simulink model "Skematik_Pagi_R2024b0x2Daziz"  (R2024b)
settings: Solver=ode23tb  StartTime=0.0  StopTime=2  RelTol=1e-3
undefined symbols (not defined in the file): D1, Delta
libraries: spsThreePhaseBreakerLib x87, spsThreePhaseParallelRLCLoadLib x19, spsThreePhaseTransformerTwoWindingsLib x18, spsThreePhasePISectionLineLib x18, spsExcitationSystemLib x4, spsSynchronousMachinepuStandardLib x4, spsThreePhaseVIMeasurementLib x4, spsMultimeterLib x1, spspowerguiLib x1
settings Model: Creator=Rafi Ananta Alden  LastModifiedBy=Ahmad Aziz

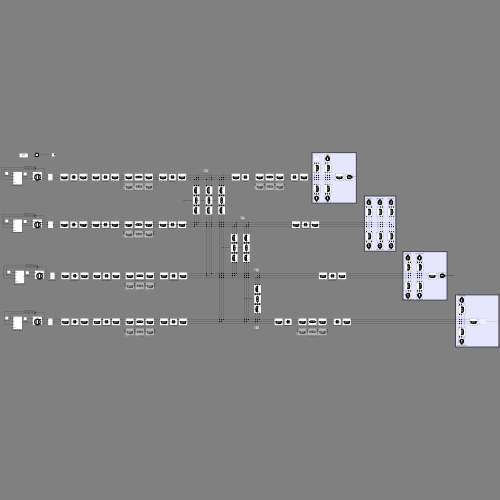
[thumbnail: Simulink's stored preview of the top-level diagram]
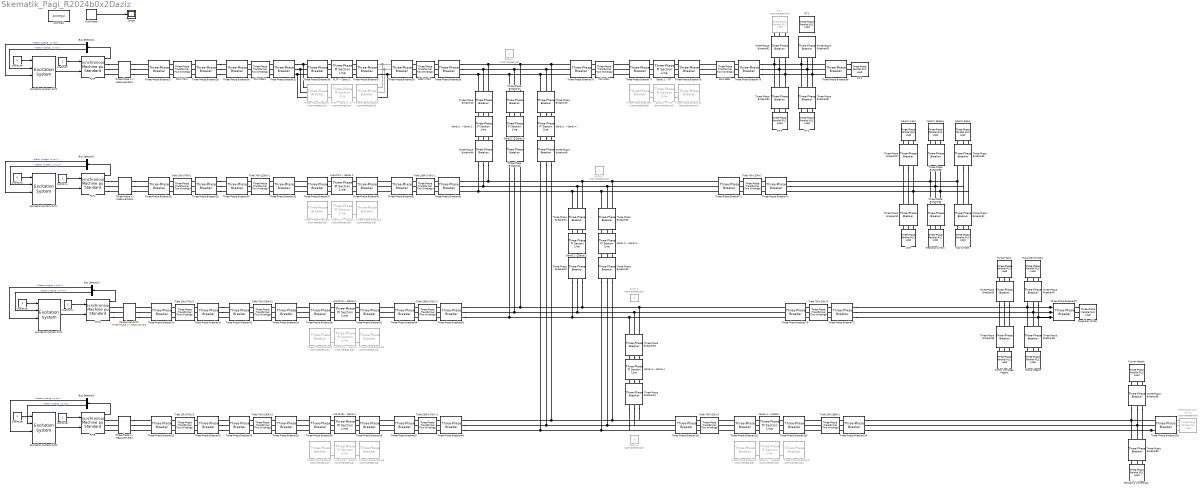
== system Skematik_Pagi_R2024b0x2Daziz ==
  20kV/380V : spsThreePhaseTransformerTwoWindingsLib/Three-Phase Transformer (Two Windings)  Winding1Connection=Yg  Winding2Connection=Delta (D1)  CoreType=Three single-phase transformers  SetSaturation=off  Hysteresis=off  DataFile='hysteresis'  SetInitialFlux=off  Measurements=None  UNITS=pu  NominalPower=[ 1000e6 , 50 ]  Winding1=[ 20e3 , 5e-3 , 0.1/(100*pi) ]  Winding2=[ 380 , 5e-3 , 0 ]  Rm=500  Lm=500  L0=0.5  Saturation=[ 0,0 ; 0.0024,1.2 ; 1.0,1.52 ]  InitialFluxes=[ 0.8 , -0.8 , 0.7 ]  BreakLoop=off  DiscreteSolver=Trapezoidal iterative  DataType=off  TransfoNumber=1
  20kV/70kV : spsThreePhaseTransformerTwoWindingsLib/Three-Phase Transformer (Two Windings)  Winding1Connection=Yg  Winding2Connection=Delta (D1)  CoreType=Three single-phase transformers  SetSaturation=off  Hysteresis=off  DataFile='hysteresis'  SetInitialFlux=off  Measurements=None  UNITS=pu  NominalPower=[ 250e6 , 50 ]  Winding1=[ 20e3 , 0.005 , 0 ]  Winding2=[ 70e3 , 0.005 , 0.1/314 ]  Rm=500  Lm=500  L0=0.5  Saturation=[ 0,0 ; 0.0024,1.2 ; 1.0,1.52 ]  InitialFluxes=[ 0.8 , -0.8 , 0.7 ]  BreakLoop=off  DiscreteSolver=Trapezoidal iterative  DataType=off  TransfoNumber=1
  "230kV/70kV " : spsThreePhaseTransformerTwoWindingsLib/Three-Phase Transformer (Two Windings)  Winding1Connection=Yg  Winding2Connection=Delta (D1)  CoreType=Three single-phase transformers  SetSaturation=off  Hysteresis=off  DataFile='hysteresis'  SetInitialFlux=off  Measurements=None  UNITS=pu  NominalPower=[ 250e6 , 50 ]  Winding1=[ 230e3 , 5e-3 , 0.1/(100*pi) ]  Winding2=[ 70e3 , 5e-3 , 0 ]  Rm=500  Lm=500  L0=0.5  Saturation=[ 0,0 ; 0.0024,1.2 ; 1.0,1.52 ]  InitialFluxes=[ 0.8 , -0.8 , 0.7 ]  BreakLoop=off  DiscreteSolver=Trapezoidal iterative  DataType=off  TransfoNumber=1
  70kV/20kV : spsThreePhaseTransformerTwoWindingsLib/Three-Phase Transformer (Two Windings)  Winding1Connection=Delta (D1)  Winding2Connection=Yg  CoreType=Three single-phase transformers  SetSaturation=off  Hysteresis=off  DataFile='hysteresis'  SetInitialFlux=off  Measurements=None  UNITS=pu  NominalPower=[ 250e6 , 50 ]  Winding1=[70e3 , 0.005 , 0.1/314 ]  Winding2=[ 20e3 , 0.005 , 0 ]  Rm=500  Lm=500  L0=0.5  Saturation=[ 0,0 ; 0.0024,1.2 ; 1.0,1.52 ]  InitialFluxes=[ 0.8 , -0.8 , 0.7 ]  BreakLoop=off  DiscreteSolver=Trapezoidal iterative  DataType=off  TransfoNumber=1
  70kV/230kV : spsThreePhaseTransformerTwoWindingsLib/Three-Phase Transformer (Two Windings)  Winding1Connection=Delta (D1)  Winding2Connection=Yg  CoreType=Three single-phase transformers  SetSaturation=off  Hysteresis=off  DataFile='hysteresis'  SetInitialFlux=off  Measurements=None  UNITS=pu  NominalPower=[ 250e6 , 50 ]  Winding1=[ 70e3 , 5e-3 , 0.1/(100*pi) ]  Winding2=[ 230e3 , 5e-3 , 0 ]  Rm=500  Lm=500  L0=0.5  Saturation=[ 0,0 ; 0.0024,1.2 ; 1.0,1.52 ]  InitialFluxes=[ 0.8 , -0.8 , 0.7 ]  BreakLoop=off  DiscreteSolver=Trapezoidal iterative  DataType=off  TransfoNumber=1
  Bus Selector{1..4} (4 alike) : BusSelector  OutputSignals="dq0 components.Stator voltage  vq (pu),dq0 components.Stator voltage  vd (pu)"
  Excitation System PLTA : spsExcitationSystemLib/Excitation System  tr=20e-3  reg=[ 300, 0.001 ]  exc=[ 1, 0 ]  tgr=[ 0, 0 ]  damp=[ 0.001, 0.1 ]  sat=[ 0, 0 ]  lim=[ -11.5, 11.5, 0 ]  v0="[1.0  1.28]"
      settings: LibrarySourceBlock=sps_lib/Electrical Machines/Synchronous Machine Control/Excitation System
  Excitation System PLTB : spsExcitationSystemLib/Excitation System  tr=20e-3  reg=[ 300, 0.001 ]  exc=[ 1, 0 ]  tgr=[ 0, 0 ]  damp=[ 0.001, 0.1 ]  sat=[ 0, 0 ]  lim=[ -11.5, 11.5, 0 ]  v0="[1.0  1.28]"
      settings: LibrarySourceBlock=sps_lib/Electrical Machines/Synchronous Machine Control/Excitation System
  Excitation System PLTP : spsExcitationSystemLib/Excitation System  tr=20e-3  reg=[ 300, 0.001 ]  exc=[ 1, 0 ]  tgr=[ 0, 0 ]  damp=[ 0.001, 0.1 ]  sat=[ 0, 0 ]  lim=[ -11.5, 11.5, 0 ]  v0="[1.0  1.28]"
      settings: LibrarySourceBlock=sps_lib/Electrical Machines/Synchronous Machine Control/Excitation System
  Excitation System PLTU : spsExcitationSystemLib/Excitation System  tr=20e-3  reg=[ 300, 0.001 ]  exc=[ 1, 0 ]  tgr=[ 0, 0 ]  damp=[ 0.001, 0.1 ]  sat=[ 0, 0 ]  lim=[ -11.5, 11.5, 0 ]  v0="[1.0  1.28]"
      settings: LibrarySourceBlock=sps_lib/Electrical Machines/Synchronous Machine Control/Excitation System
  Gardu 1 : Constant  Commented=on
  "Gardu 1 -- Gardu 2" : spsThreePhasePISectionLineLib/Three-Phase PI Section Line  LConnTagsString=a|b|c  RConnTagsString=A|B|C  Length=20  Frequency=50  Resistances=[ 0.2 0.2]  Inductances="[ 0.00637  0.00637]"  Capacitances=[12.74e-9 7.751e-9]
  "Gardu 1 -- Gardu 3" : spsThreePhasePISectionLineLib/Three-Phase PI Section Line  LConnTagsString=a|b|c  RConnTagsString=A|B|C  Length=5  Frequency=50  Resistances=[ 0.2 0.2]  Inductances="[ 0.00637  0.00637]"  Capacitances=[12.74e-9 7.751e-9]
  "Gardu 1 -- Gardu 4" : spsThreePhasePISectionLineLib/Three-Phase PI Section Line  LConnTagsString=a|b|c  RConnTagsString=A|B|C  Length=20  Frequency=50  Resistances=[ 0.2 0.2]  Inductances="[ 0.00637  0.00637]"  Capacitances=[12.74e-9 7.751e-9]
  "Gardu 1 -- RT" : spsThreePhasePISectionLineLib/Three-Phase PI Section Line  LConnTagsString=a|b|c  RConnTagsString=A|B|C  Length=3  Frequency=50  Resistances=[ 0.2 0.2]  Inductances="[ 0.00637  0.00637]"  Capacitances=[12.74e-9 7.751e-9]
  "Gardu 1 -- RT1" : spsThreePhasePISectionLineLib/Three-Phase PI Section Line  Commented=on  LConnTagsString=a|b|c  RConnTagsString=A|B|C  Length=3  Frequency=50  Resistances=[0.05 0.25]  Inductances=[0.001 0.003]  Capacitances=[10e-9 7e-9]
  Gardu 2 : Constant  Commented=on  Value=2
  "Gardu 2 -- Gardu 3" : spsThreePhasePISectionLineLib/Three-Phase PI Section Line  LConnTagsString=a|b|c  RConnTagsString=A|B|C  Length=5  Frequency=50  Resistances=[ 0.2 0.2]  Inductances="[ 0.00637  0.00637]"  Capacitances=[12.74e-9 7.751e-9]
  "Gardu 2 -- Gardu 4" : spsThreePhasePISectionLineLib/Three-Phase PI Section Line  LConnTagsString=a|b|c  RConnTagsString=A|B|C  Length=20  Frequency=50  Resistances=[ 0.2 0.2]  Inductances="[ 0.00637  0.00637]"  Capacitances=[12.74e-9 7.751e-9]
  Gardu 3 : Constant  Commented=on  Value=3
  "Gardu 3 -- Gardu 4" : spsThreePhasePISectionLineLib/Three-Phase PI Section Line  LConnTagsString=a|b|c  RConnTagsString=A|B|C  Length=5  Frequency=50  Resistances=[ 0.2 0.2]  Inductances="[ 0.00637  0.00637]"  Capacitances=[12.74e-9 7.751e-9]
  Gardu 4 : Constant  Commented=on  Value=4
  "Gardu 4 -- PubSos" : spsThreePhasePISectionLineLib/Three-Phase PI Section Line  LConnTagsString=a|b|c  RConnTagsString=A|B|C  Length=3  Frequency=50  Resistances=[ 0.1 0.1]  Inductances="[ 0.00637  0.00637]"  Capacitances=[12.74e-9 7.751e-9]
  "Gardu 4 -- PubSos1" : spsThreePhasePISectionLineLib/Three-Phase PI Section Line  Commented=on  LConnTagsString=a|b|c  RConnTagsString=A|B|C  Length=3  Frequency=50  Resistances=[0.05 0.25]  Inductances=[0.001 0.003]  Capacitances=[10e-9 7e-9]
  Industri Besar : spsThreePhaseParallelRLCLoadLib/Three-Phase Parallel RLC Load  LConnTagsString=A|B|C  Configuration=Y (grounded)  NominalVoltage=20e3  Vabc=[1e3 1e3 1e3]  Vabcp=[1e3 1e3 1e3]  NominalFrequency=50  UnbalancedPower=off  ActivePower=9.00e6  InductivePower=4.36e6  CapacitivePower=0  Pabc=[10e3 9e3 11e3]  QLabc=[100 90 110]  QCabc=[100 90 110]  Pabcp=[10e3 9e3 11e3]  QLabcp=[100 90 110]  QCabcp=[100 90 110]  Measurements=Branch voltages and currents  LoadType=constant Z
  Industri Kecil : spsThreePhaseParallelRLCLoadLib/Three-Phase Parallel RLC Load  LConnTagsString=A|B|C  Configuration=Y (grounded)  NominalVoltage=20e3  Vabc=[1e3 1e3 1e3]  Vabcp=[1e3 1e3 1e3]  NominalFrequency=50  UnbalancedPower=off  ActivePower=5.94e9  InductivePower=2.88e9  CapacitivePower=0  Pabc=[10e3 9e3 11e3]  QLabc=[100 90 110]  QCabc=[100 90 110]  Pabcp=[10e3 9e3 11e3]  QLabcp=[100 90 110]  QCabcp=[100 90 110]  Measurements=Branch voltages and currents  LoadType=constant Z
  Industri Sedang : spsThreePhaseParallelRLCLoadLib/Three-Phase Parallel RLC Load  LConnTagsString=A|B|C  Configuration=Y (grounded)  NominalVoltage=20e3  Vabc=[1e3 1e3 1e3]  Vabcp=[1e3 1e3 1e3]  NominalFrequency=50  UnbalancedPower=off  ActivePower=4.50e7  InductivePower=2.18e7  CapacitivePower=0  Pabc=[10e3 9e3 11e3]  QLabc=[100 90 110]  QCabc=[100 90 110]  Pabcp=[10e3 9e3 11e3]  QLabcp=[100 90 110]  QCabcp=[100 90 110]  Measurements=Branch voltages and currents  LoadType=constant Z
  Istana Negara : spsThreePhaseParallelRLCLoadLib/Three-Phase Parallel RLC Load  LConnTagsString=A|B|C  Configuration=Y (grounded)  NominalVoltage=20e3  Vabc=[1e3 1e3 1e3]  Vabcp=[1e3 1e3 1e3]  NominalFrequency=50  UnbalancedPower=off  ActivePower=1.17e6  InductivePower=5.67e5  CapacitivePower=0  Pabc=[10e3 9e3 11e3]  QLabc=[100 90 110]  QCabc=[100 90 110]  Pabcp=[10e3 9e3 11e3]  QLabcp=[100 90 110]  QCabcp=[100 90 110]  Measurements=Branch voltages and currents  LoadType=constant Z
  Kantor Lembaga Negara : spsThreePhaseParallelRLCLoadLib/Three-Phase Parallel RLC Load  LConnTagsString=A|B|C  Configuration=Y (grounded)  NominalVoltage=20e3  Vabc=[1e3 1e3 1e3]  Vabcp=[1e3 1e3 1e3]  NominalFrequency=50  UnbalancedPower=off  ActivePower=1.80e6  InductivePower=8.72e5  CapacitivePower=0  Pabc=[10e3 9e3 11e3]  QLabc=[100 90 110]  QCabc=[100 90 110]  Pabcp=[10e3 9e3 11e3]  QLabcp=[100 90 110]  QCabcp=[100 90 110]  Measurements=Branch voltages and currents  LoadType=constant Z
  "Line PLTA -- Gardu 1" : spsThreePhasePISectionLineLib/Three-Phase PI Section Line  Commented=on  LConnTagsString=a|b|c  RConnTagsString=A|B|C  Length=50  Frequency=50  Resistances=[ 0.2 0.3864]  Inductances="[ 2/(100*pi)  4.1264e-3]"  Capacitances=[12.74e-9 7.751e-9]
  "Line PLTA -- Gardu 3" : spsThreePhasePISectionLineLib/Three-Phase PI Section Line  LConnTagsString=a|b|c  RConnTagsString=A|B|C  Length=50  Frequency=50  Resistances=[ 0.2 0.3864]  Inductances="[ 2/(100*pi)  4.1264e-3]"  Capacitances=[12.74e-9 7.751e-9]
  "Line PLTB -- Gardu 1" : spsThreePhasePISectionLineLib/Three-Phase PI Section Line  Commented=on  LConnTagsString=a|b|c  RConnTagsString=A|B|C  Length=20  Frequency=50  Resistances=[ 0.2 0.3864]  Inductances="[ 2/(100*pi)  4.1264e-3]"  Capacitances=[12.74e-9 7.751e-9]
  "Line PLTB -- Gardu 4" : spsThreePhasePISectionLineLib/Three-Phase PI Section Line  LConnTagsString=a|b|c  RConnTagsString=A|B|C  Length=20  Frequency=50  Resistances=[ 0.2 0.3864]  Inductances="[ 2/(100*pi)  4.1264e-3]"  Capacitances=[12.74e-9 7.751e-9]
  "Line PLTU -- Gardu 1" : spsThreePhasePISectionLineLib/Three-Phase PI Section Line  Commented=on  LConnTagsString=a|b|c  RConnTagsString=A|B|C  Length=100  Frequency=50  Resistances=[0.05 0.25]  Inductances=[0.001 0.003]  Capacitances=[10e-9 7e-9]
  "Line PLTU -- Gardu 2" : spsThreePhasePISectionLineLib/Three-Phase PI Section Line  LConnTagsString=a|b|c  RConnTagsString=A|B|C  Length=100  Frequency=50  Resistances=[ 0.2 0.2]  Inductances="[ 0.00637  0.00637]"  Capacitances=[12.74e-9 7.751e-9]
  Mall & Hotel : spsThreePhaseParallelRLCLoadLib/Three-Phase Parallel RLC Load  LConnTagsString=A|B|C  Configuration=Y (grounded)  NominalVoltage=20e3  Vabc=[1e3 1e3 1e3]  Vabcp=[1e3 1e3 1e3]  NominalFrequency=50  UnbalancedPower=off  ActivePower=9.00e5  InductivePower=4.36e5  CapacitivePower=0  Pabc=[10e3 9e3 11e3]  QLabc=[100 90 110]  QCabc=[100 90 110]  Pabcp=[10e3 9e3 11e3]  QLabcp=[100 90 110]  QCabcp=[100 90 110]  Measurements=Branch voltages and currents  LoadType=constant Z
  Multimeter : spsMultimeterLib/Multimeter  L=108  sel=1  yselected={}  Gain=0  OutputType=Magnitude  PlotAtSimulationStop=off  PhasorSimulation=on
  PLTA : spsSynchronousMachinepuStandardLib/Synchronous Machine pu Standard  PresetModel=No  MechanicalLoad=Mechanical power Pm  ShowDetailedParameters=on  RotorType=Salient-pole  Units=per unit standard parameters  MeasurementBus=off  NominalParameters="[34e6  20e3   50]"  Reactances1=[ 1.81, 0.3, 0.23, 1.76, 0.65, 0.25, 0.15 ]  Reactances2="[1.305, 0.296, 0.252, 0.474,  0.243,  0.1]"  dAxisTimeConstants=Open-circuit  qAxisTimeConstants=Short-circuit  TimeConstants1="[ 4.4849  0.0681  0.1  ]"  TimeConstants2=[ 8.0, 0.03, 1.0, 0.07 ]  TimeConstants3="[  4.49  0.0681  0.0513  ]"  TimeConstants4=[ 8.0, 0.03, 0.3371, 0.0295 ]  TimeConstants5=[ 1.01, 0.053, 0.1 ]  TimeConstants6=[ 1.3201, 0.023, 1.0, 0.07 ]  TimeConstants7=[0.012 0.003 0.003]  TimeConstants8=[ 1.3201, 0.0231, 0.3371, 0.0295 ]  StatorResistance=0.003  Mechanical=[3.7 0 20]  PolePairs=20  InitialConditions=[0 -84.041 0.282629 0.282629 0.282629 44.9561 -75.0439 164.956 0.763822]  SetSaturation=off  Saturation=[0.6404,0.7127,0.8441,0.9214,0.9956,1.082,1.19,1.316,1.457;0.7,0.7698,0.8872,0.9466,0.9969,1.046,1.1,1.151,1.201]  LoadFlowParameters=[1,0,0,0,0]  TsPowergui=0  TsBlock=-1  IterativeModel=Trapezoidal non iterative  IterativeDiscreteModel=Trapezoidal non iterative  BusType=swing  Pref=100e6*1  Qref=0  Qmin=-100e6  Qmax=100e6  PLF=0  QLF=0
  PLTB : spsSynchronousMachinepuStandardLib/Synchronous Machine pu Standard  PresetModel=No  MechanicalLoad=Mechanical power Pm  ShowDetailedParameters=on  RotorType=Salient-pole  Units=per unit standard parameters  MeasurementBus=off  NominalParameters="[11e6  20e3   50]"  Reactances1=[ 1.81, 0.3, 0.23, 1.76, 0.65, 0.25, 0.15 ]  Reactances2="[1.305, 0.296, 0.252, 0.474,  0.243,  0.1]"  dAxisTimeConstants=Open-circuit  qAxisTimeConstants=Short-circuit  TimeConstants1="[ 4.4849  0.0681  0.1  ]"  TimeConstants2=[ 8.0, 0.03, 1.0, 0.07 ]  TimeConstants3="[  4.49  0.0681  0.0513  ]"  TimeConstants4=[ 8.0, 0.03, 0.3371, 0.0295 ]  TimeConstants5=[ 1.01, 0.053, 0.1 ]  TimeConstants6=[ 1.3201, 0.023, 1.0, 0.07 ]  TimeConstants7=[0.012 0.003 0.003]  TimeConstants8=[ 1.3201, 0.0231, 0.3371, 0.0295 ]  StatorResistance=0.003  Mechanical=[3.7 0 20]  PolePairs=20  InitialConditions=[0 -84.041 0.282629 0.282629 0.282629 44.9561 -75.0439 164.956 0.763822]  SetSaturation=off  Saturation=[0.6404,0.7127,0.8441,0.9214,0.9956,1.082,1.19,1.316,1.457;0.7,0.7698,0.8872,0.9466,0.9969,1.046,1.1,1.151,1.201]  LoadFlowParameters=[1,0,0,0,0]  TsPowergui=0  TsBlock=-1  IterativeModel=Trapezoidal non iterative  IterativeDiscreteModel=Trapezoidal non iterative  BusType=PV  Pref=100e6*1  Qref=0  Qmin=-100e6  Qmax=100e6  PLF=0  QLF=0
  "PLTP " : spsSynchronousMachinepuStandardLib/Synchronous Machine pu Standard  PresetModel=No  MechanicalLoad=Mechanical power Pm  ShowDetailedParameters=on  RotorType=Salient-pole  Units=per unit standard parameters  MeasurementBus=off  NominalParameters="[89e6  20e3   50]"  Reactances1=[ 1.81, 0.3, 0.23, 1.76, 0.65, 0.25, 0.15 ]  Reactances2="[1.305, 0.296, 0.252, 0.474,  0.243,  0.1]"  dAxisTimeConstants=Open-circuit  qAxisTimeConstants=Short-circuit  TimeConstants1="[ 4.4849  0.0681  0.1  ]"  TimeConstants2=[ 8.0, 0.03, 1.0, 0.07 ]  TimeConstants3="[  4.49  0.0681  0.0513  ]"  TimeConstants4=[ 8.0, 0.03, 0.3371, 0.0295 ]  TimeConstants5=[ 1.01, 0.053, 0.1 ]  TimeConstants6=[ 1.3201, 0.023, 1.0, 0.07 ]  TimeConstants7=[0.012 0.003 0.003]  TimeConstants8=[ 1.3201, 0.0231, 0.3371, 0.0295 ]  StatorResistance=0.003  Mechanical=[3.7 0 20]  PolePairs=20  InitialConditions=[0 -87.2037 0.333145 0.333145 0.333145 75.164 -44.836 195.164 0.584783]  SetSaturation=off  Saturation=[0.6404,0.7127,0.8441,0.9214,0.9956,1.082,1.19,1.316,1.457;0.7,0.7698,0.8872,0.9466,0.9969,1.046,1.1,1.151,1.201]  LoadFlowParameters=[1,0,0,0,0]  TsPowergui=0  TsBlock=-1  IterativeModel=Trapezoidal non iterative  IterativeDiscreteModel=Trapezoidal non iterative  BusType=swing  Pref=0  Qref=0  Qmin=-inf  Qmax=inf  PLF=0  QLF=0
  "PLTP -- Gardu 1" : spsThreePhasePISectionLineLib/Three-Phase PI Section Line  LConnTagsString=a|b|c  RConnTagsString=A|B|C  Length=100  Frequency=50  Resistances=[ 0.2 0.2]  Inductances="[ 0.00637  0.00637]"  Capacitances=[12.74e-9 7.751e-9]
  "PLTP -- Gardu 1 (1)" : spsThreePhasePISectionLineLib/Three-Phase PI Section Line  Commented=on  LConnTagsString=a|b|c  RConnTagsString=A|B|C  Length=100  Frequency=50  Resistances=[0.05 0.25]  Inductances=[0.001 0.003]  Capacitances=[10e-9 7e-9]
  PLTU : spsSynchronousMachinepuStandardLib/Synchronous Machine pu Standard  PresetModel=No  MechanicalLoad=Mechanical power Pm  ShowDetailedParameters=on  RotorType=Salient-pole  Units=per unit standard parameters  MeasurementBus=off  NominalParameters="[111e6  20e3   50]"  Reactances1=[ 1.81, 0.3, 0.23, 1.76, 0.65, 0.25, 0.15 ]  Reactances2="[1.305, 0.296, 0.252, 0.474,  0.243,  0.1]"  dAxisTimeConstants=Open-circuit  qAxisTimeConstants=Short-circuit  TimeConstants1="[ 4.4849  0.0681  0.1  ]"  TimeConstants2=[ 8.0, 0.03, 1.0, 0.07 ]  TimeConstants3="[  4.49  0.0681  0.0513  ]"  TimeConstants4=[ 8.0, 0.03, 0.3371, 0.0295 ]  TimeConstants5=[ 1.01, 0.053, 0.1 ]  TimeConstants6=[ 1.3201, 0.023, 1.0, 0.07 ]  TimeConstants7=[0.012 0.003 0.003]  TimeConstants8=[ 1.3201, 0.0231, 0.3371, 0.0295 ]  StatorResistance=0.003  Mechanical=[3.7 0 20]  PolePairs=20  InitialConditions=[0 -84.041 0.282629 0.282629 0.282629 44.9561 -75.0439 164.956 0.763822]  SetSaturation=off  Saturation=[0.6404,0.7127,0.8441,0.9214,0.9956,1.082,1.19,1.316,1.457;0.7,0.7698,0.8872,0.9466,0.9969,1.046,1.1,1.151,1.201]  LoadFlowParameters=[1,0,0,0,0]  TsPowergui=0  TsBlock=-1  IterativeModel=Trapezoidal non iterative  IterativeDiscreteModel=Trapezoidal non iterative  BusType=PV  Pref=82e6  Qref=0  Qmin=-100e6  Qmax=100e6  PLF=0  QLF=0
  Pangkalan Militer : spsThreePhaseParallelRLCLoadLib/Three-Phase Parallel RLC Load  LConnTagsString=A|B|C  Configuration=Y (grounded)  NominalVoltage=20e3  Vabc=[1e3 1e3 1e3]  Vabcp=[1e3 1e3 1e3]  NominalFrequency=50  UnbalancedPower=off  ActivePower=1.35e4  InductivePower=6.54e3  CapacitivePower=0  Pabc=[10e3 9e3 11e3]  QLabc=[100 90 110]  QCabc=[100 90 110]  Pabcp=[10e3 9e3 11e3]  QLabcp=[100 90 110]  QCabcp=[100 90 110]  Measurements=Branch voltages and currents  LoadType=constant Z
  Penerangan Jalan Umum : spsThreePhaseParallelRLCLoadLib/Three-Phase Parallel RLC Load  Commented=on  LConnTagsString=A|B|C  Configuration=Y (grounded)  NominalVoltage=20e3  Vabc=[1e3 1e3 1e3]  Vabcp=[1e3 1e3 1e3]  NominalFrequency=50  UnbalancedPower=off  ActivePower=0  InductivePower=0  CapacitivePower=0  Pabc=[10e3 9e3 11e3]  QLabc=[100 90 110]  QCabc=[100 90 110]  Pabcp=[10e3 9e3 11e3]  QLabcp=[100 90 110]  QCabcp=[100 90 110]  Measurements=Branch voltages and currents  LoadType=constant Z
  Pengukuran PLTA : spsThreePhaseVIMeasurementLib/Three-Phase V-I Measurement  VoltageMeasurement=phase-to-ground  SetLabelV=on  LabelV=V_PLTA  Vpu=off  VpuLL=off  CurrentMeasurement=yes  SetLabelI=on  LabelI=I_PLTA  Ipu=off  Pbase=100e6  Vbase=500e3  OutputType=Complex  PhasorSimulation=on  PSBequivalent=0
  Pref PLTA : Constant
  Pref PLTB : Constant
  Pref PLTP : Constant
  Pref PLTU : Constant
  Pusat Server Data : spsThreePhaseParallelRLCLoadLib/Three-Phase Parallel RLC Load  LConnTagsString=A|B|C  Configuration=Y (grounded)  NominalVoltage=20e3  Vabc=[1e3 1e3 1e3]  Vabcp=[1e3 1e3 1e3]  NominalFrequency=50  UnbalancedPower=off  ActivePower=2.25e5  InductivePower=1.09e5  CapacitivePower=0  Pabc=[10e3 9e3 11e3]  QLabc=[100 90 110]  QCabc=[100 90 110]  Pabcp=[10e3 9e3 11e3]  QLabcp=[100 90 110]  QCabcp=[100 90 110]  Measurements=Branch voltages and currents  LoadType=constant Z
  RT 1 : spsThreePhaseParallelRLCLoadLib/Three-Phase Parallel RLC Load  Commented=on  LConnTagsString=A|B|C  Configuration=Y (grounded)  NominalVoltage=20e3  Vabc=[1e3 1e3 1e3]  Vabcp=[1e3 1e3 1e3]  NominalFrequency=50  UnbalancedPower=off  ActivePower=0  InductivePower=0  CapacitivePower=0  Pabc=[10e3 9e3 11e3]  QLabc=[100 90 110]  QCabc=[100 90 110]  Pabcp=[10e3 9e3 11e3]  QLabcp=[100 90 110]  QCabcp=[100 90 110]  Measurements=Branch voltages and currents  LoadType=constant Z
  RT 2 : spsThreePhaseParallelRLCLoadLib/Three-Phase Parallel RLC Load  LConnTagsString=A|B|C  Configuration=Y (grounded)  NominalVoltage=20e3  Vabc=[1e3 1e3 1e3]  Vabcp=[1e3 1e3 1e3]  NominalFrequency=50  UnbalancedPower=off  ActivePower=8e6  InductivePower=3.87e6  CapacitivePower=0  Pabc=[10e3 9e3 11e3]  QLabc=[100 90 110]  QCabc=[100 90 110]  Pabcp=[10e3 9e3 11e3]  QLabcp=[100 90 110]  QCabcp=[100 90 110]  Measurements=Branch voltages and currents  LoadType=constant Z
  RT 3 : spsThreePhaseParallelRLCLoadLib/Three-Phase Parallel RLC Load  LConnTagsString=A|B|C  Configuration=Y (grounded)  NominalVoltage=20e3  Vabc=[1e3 1e3 1e3]  Vabcp=[1e3 1e3 1e3]  NominalFrequency=50  UnbalancedPower=off  ActivePower=5.10e6  InductivePower=2.47e6  CapacitivePower=0  Pabc=[10e3 9e3 11e3]  QLabc=[100 90 110]  QCabc=[100 90 110]  Pabcp=[10e3 9e3 11e3]  QLabcp=[100 90 110]  QCabcp=[100 90 110]  Measurements=Branch voltages and currents  LoadType=constant Z
  RT 4 : spsThreePhaseParallelRLCLoadLib/Three-Phase Parallel RLC Load  LConnTagsString=A|B|C  Configuration=Y (grounded)  NominalVoltage=20e3  Vabc=[1e3 1e3 1e3]  Vabcp=[1e3 1e3 1e3]  NominalFrequency=50  UnbalancedPower=off  ActivePower=2.10e6  InductivePower=1.02e6  CapacitivePower=0  Pabc=[10e3 9e3 11e3]  QLabc=[100 90 110]  QCabc=[100 90 110]  Pabcp=[10e3 9e3 11e3]  QLabcp=[100 90 110]  QCabcp=[100 90 110]  Measurements=Branch voltages and currents  LoadType=constant Z
  RT 5 : spsThreePhaseParallelRLCLoadLib/Three-Phase Parallel RLC Load  LConnTagsString=A|B|C  Configuration=Y (grounded)  NominalVoltage=20e3  Vabc=[1e3 1e3 1e3]  Vabcp=[1e3 1e3 1e3]  NominalFrequency=50  UnbalancedPower=off  ActivePower=3.60e6  InductivePower=1.74e6  CapacitivePower=0  Pabc=[10e3 9e3 11e3]  QLabc=[100 90 110]  QCabc=[100 90 110]  Pabcp=[10e3 9e3 11e3]  QLabcp=[100 90 110]  QCabcp=[100 90 110]  Measurements=Branch voltages and currents  LoadType=constant Z
  Restoran & Toko : spsThreePhaseParallelRLCLoadLib/Three-Phase Parallel RLC Load  LConnTagsString=A|B|C  Configuration=Y (grounded)  NominalVoltage=20e3  Vabc=[1e3 1e3 1e3]  Vabcp=[1e3 1e3 1e3]  NominalFrequency=50  UnbalancedPower=off  ActivePower=4.50e6  InductivePower=2.18e6  CapacitivePower=0  Pabc=[10e3 9e3 11e3]  QLabc=[100 90 110]  QCabc=[100 90 110]  Pabcp=[10e3 9e3 11e3]  QLabcp=[100 90 110]  QCabcp=[100 90 110]  Measurements=Branch voltages and currents  LoadType=constant Z
  Rumah Ibadah : spsThreePhaseParallelRLCLoadLib/Three-Phase Parallel RLC Load  LConnTagsString=A|B|C  Configuration=Y (grounded)  NominalVoltage=20e3  Vabc=[1e3 1e3 1e3]  Vabcp=[1e3 1e3 1e3]  NominalFrequency=50  UnbalancedPower=off  ActivePower=5.94e9  InductivePower=2.88e9  CapacitivePower=0  Pabc=[10e3 9e3 11e3]  QLabc=[100 90 110]  QCabc=[100 90 110]  Pabcp=[10e3 9e3 11e3]  QLabcp=[100 90 110]  QCabcp=[100 90 110]  Measurements=Branch voltages and currents  LoadType=constant Z
  Rumah Sakit : spsThreePhaseParallelRLCLoadLib/Three-Phase Parallel RLC Load  LConnTagsString=A|B|C  Configuration=Y (grounded)  NominalVoltage=20e3  Vabc=[1e3 1e3 1e3]  Vabcp=[1e3 1e3 1e3]  NominalFrequency=50  UnbalancedPower=off  ActivePower=3.96e7  InductivePower=1.92e7  CapacitivePower=0  Pabc=[10e3 9e3 11e3]  QLabc=[100 90 110]  QCabc=[100 90 110]  Pabcp=[10e3 9e3 11e3]  QLabcp=[100 90 110]  QCabcp=[100 90 110]  Measurements=Branch voltages and currents  LoadType=constant Z
  Scope : Scope
  Sekolah & Universitas : spsThreePhaseParallelRLCLoadLib/Three-Phase Parallel RLC Load  LConnTagsString=A|B|C  Configuration=Y (grounded)  NominalVoltage=20e3  Vabc=[1e3 1e3 1e3]  Vabcp=[1e3 1e3 1e3]  NominalFrequency=50  UnbalancedPower=off  ActivePower=4.50e7  InductivePower=2.18e7  CapacitivePower=0  Pabc=[10e3 9e3 11e3]  QLabc=[100 90 110]  QCabc=[100 90 110]  Pabcp=[10e3 9e3 11e3]  QLabcp=[100 90 110]  QCabcp=[100 90 110]  Measurements=Branch voltages and currents  LoadType=constant Z
  Three-Phase V-I Measurement1 : spsThreePhaseVIMeasurementLib/Three-Phase V-I Measurement  VoltageMeasurement=phase-to-ground  SetLabelV=on  LabelV=V_PLTU  Vpu=off  VpuLL=off  CurrentMeasurement=yes  SetLabelI=on  LabelI=I_PLTU  Ipu=off  Pbase=100e6  Vbase=500e3  OutputType=Magnitude  PhasorSimulation=on  PSBequivalent=0
  Three-Phase V-I Measurement2 : spsThreePhaseVIMeasurementLib/Three-Phase V-I Measurement  VoltageMeasurement=phase-to-ground  SetLabelV=on  LabelV=V_PLTB  Vpu=off  VpuLL=off  CurrentMeasurement=yes  SetLabelI=on  LabelI=I_PLTB  Ipu=off  Pbase=100e6  Vbase=500e3  OutputType=Complex  PhasorSimulation=on  PSBequivalent=0
  Three-Phase V-I Measurement4 : spsThreePhaseVIMeasurementLib/Three-Phase V-I Measurement  VoltageMeasurement=phase-to-ground  SetLabelV=on  LabelV=V_PLTP  Vpu=off  VpuLL=off  CurrentMeasurement=yes  SetLabelI=on  LabelI=I_PLTP  Ipu=off  Pbase=100e6  Vbase=500e3  OutputType=Complex  PhasorSimulation=on  PSBequivalent=0
  Three-Phase Breaker{1..12} (12 alike) : spsThreePhaseBreakerLib/Three-Phase Breaker  Commented=on  InitialState=closed  SwitchA=on  SwitchB=on  SwitchC=on  SwitchTimes="[0.4  1.3]"  External=off  BreakerResistance=0.01  SnubberResistance=1e6  SnubberCapacitance=inf  Measurements=None
  Three-Phase Breaker{24..67,70..73,76..79,82..104} (75 alike) : spsThreePhaseBreakerLib/Three-Phase Breaker  InitialState=closed  SwitchA=on  SwitchB=on  SwitchC=on  SwitchTimes="[0.4  1.3]"  External=off  BreakerResistance=0.01  SnubberResistance=1e6  SnubberCapacitance=inf  Measurements=None
  Trafo 20kV/380V1 : spsThreePhaseTransformerTwoWindingsLib/Three-Phase Transformer (Two Windings)  Winding1Connection=Yg  Winding2Connection=Delta (D1)  CoreType=Three single-phase transformers  SetSaturation=off  Hysteresis=off  DataFile='hysteresis'  SetInitialFlux=off  Measurements=None  UNITS=pu  NominalPower=[ 1000e6 , 50 ]  Winding1=[ 20e3 , 5e-3 , 0.1/(100*pi) ]  Winding2=[ 380 , 5e-3 , 0 ]  Rm=500  Lm=500  L0=0.5  Saturation=[ 0,0 ; 0.0024,1.2 ; 1.0,1.52 ]  InitialFluxes=[ 0.8 , -0.8 , 0.7 ]  BreakLoop=off  DiscreteSolver=Trapezoidal iterative  DataType=off  TransfoNumber=1
  Trafo 20kV/70kV1 : spsThreePhaseTransformerTwoWindingsLib/Three-Phase Transformer (Two Windings)  Winding1Connection=Yg  Winding2Connection=Delta (D1)  CoreType=Three single-phase transformers  SetSaturation=off  Hysteresis=off  DataFile='hysteresis'  SetInitialFlux=off  Measurements=None  UNITS=pu  NominalPower=[ 250e6 , 50 ]  Winding1=[ 20e3 , 0.005 , 0 ]  Winding2=[ 70e3 , 0.005 , 0.1/314 ]  Rm=500  Lm=500  L0=0.5  Saturation=[ 0,0 ; 0.0024,1.2 ; 1.0,1.52 ]  InitialFluxes=[ 0.8 , -0.8 , 0.7 ]  BreakLoop=off  DiscreteSolver=Trapezoidal iterative  DataType=off  TransfoNumber=1
  Trafo 20kV/70kV2 : spsThreePhaseTransformerTwoWindingsLib/Three-Phase Transformer (Two Windings)  Winding1Connection=Yg  Winding2Connection=Delta (D1)  CoreType=Three single-phase transformers  SetSaturation=off  Hysteresis=off  DataFile='hysteresis'  SetInitialFlux=off  Measurements=None  UNITS=pu  NominalPower=[ 250e6 , 50 ]  Winding1=[ 20e3 , 0.005 , 0 ]  Winding2=[ 70e3 , 0.005 , 0.1/314 ]  Rm=500  Lm=500  L0=0.5  Saturation=[ 0,0 ; 0.0024,1.2 ; 1.0,1.52 ]  InitialFluxes=[ 0.8 , -0.8 , 0.7 ]  BreakLoop=off  DiscreteSolver=Trapezoidal iterative  DataType=off  TransfoNumber=1
  Trafo 20kV/70kV3 : spsThreePhaseTransformerTwoWindingsLib/Three-Phase Transformer (Two Windings)  Winding1Connection=Yg  Winding2Connection=Delta (D1)  CoreType=Three single-phase transformers  SetSaturation=off  Hysteresis=off  DataFile='hysteresis'  SetInitialFlux=off  Measurements=None  UNITS=pu  NominalPower=[ 250e6 , 50 ]  Winding1=[ 20e3 , 0.005 , 0 ]  Winding2=[ 70e3 , 0.005 , 0.1/314 ]  Rm=500  Lm=500  L0=0.5  Saturation=[ 0,0 ; 0.0024,1.2 ; 1.0,1.52 ]  InitialFluxes=[ 0.8 , -0.8 , 0.7 ]  BreakLoop=off  DiscreteSolver=Trapezoidal iterative  DataType=off  TransfoNumber=1
  Trafo 230kV/70kV 1 : spsThreePhaseTransformerTwoWindingsLib/Three-Phase Transformer (Two Windings)  Winding1Connection=Yg  Winding2Connection=Delta (D1)  CoreType=Three single-phase transformers  SetSaturation=off  Hysteresis=off  DataFile='hysteresis'  SetInitialFlux=off  Measurements=None  UNITS=pu  NominalPower=[ 250e6 , 50 ]  Winding1=[ 20e3 , 5e-3 , 0.1/(100*pi) ]  Winding2=[ 70e3 , 5e-3 , 0 ]  Rm=500  Lm=500  L0=0.5  Saturation=[ 0,0 ; 0.0024,1.2 ; 1.0,1.52 ]  InitialFluxes=[ 0.8 , -0.8 , 0.7 ]  BreakLoop=off  DiscreteSolver=Trapezoidal iterative  DataType=off  TransfoNumber=1
  Trafo 230kV/70kV 2 : spsThreePhaseTransformerTwoWindingsLib/Three-Phase Transformer (Two Windings)  Winding1Connection=Yg  Winding2Connection=Delta (D1)  CoreType=Three single-phase transformers  SetSaturation=off  Hysteresis=off  DataFile='hysteresis'  SetInitialFlux=off  Measurements=None  UNITS=pu  NominalPower=[ 250e6 , 50 ]  Winding1=[ 20e3 , 5e-3 , 0.1/(100*pi) ]  Winding2=[ 70e3 , 5e-3 , 0 ]  Rm=500  Lm=500  L0=0.5  Saturation=[ 0,0 ; 0.0024,1.2 ; 1.0,1.52 ]  InitialFluxes=[ 0.8 , -0.8 , 0.7 ]  BreakLoop=off  DiscreteSolver=Trapezoidal iterative  DataType=off  TransfoNumber=1
  Trafo 230kV/70kV 3 : spsThreePhaseTransformerTwoWindingsLib/Three-Phase Transformer (Two Windings)  Winding1Connection=Yg  Winding2Connection=Delta (D1)  CoreType=Three single-phase transformers  SetSaturation=off  Hysteresis=off  DataFile='hysteresis'  SetInitialFlux=off  Measurements=None  UNITS=pu  NominalPower=[ 250e6 , 50 ]  Winding1=[ 20e3 , 5e-3 , 0.1/(100*pi) ]  Winding2=[ 70e3 , 5e-3 , 0 ]  Rm=500  Lm=500  L0=0.5  Saturation=[ 0,0 ; 0.0024,1.2 ; 1.0,1.52 ]  InitialFluxes=[ 0.8 , -0.8 , 0.7 ]  BreakLoop=off  DiscreteSolver=Trapezoidal iterative  DataType=off  TransfoNumber=1
  Trafo 70kV/20kV1 : spsThreePhaseTransformerTwoWindingsLib/Three-Phase Transformer (Two Windings)  Winding1Connection=Delta (D1)  Winding2Connection=Yg  CoreType=Three single-phase transformers  SetSaturation=off  Hysteresis=off  DataFile='hysteresis'  SetInitialFlux=off  Measurements=None  UNITS=pu  NominalPower=[ 250e6 , 50 ]  Winding1="[ 70e3  , 0.005 , 0.1/314 ]"  Winding2=[ 20e3 , 0.005 , 0 ]  Rm=500  Lm=500  L0=0.5  Saturation=[ 0,0 ; 0.0024,1.2 ; 1.0,1.52 ]  InitialFluxes=[ 0.8 , -0.8 , 0.7 ]  BreakLoop=off  DiscreteSolver=Trapezoidal iterative  DataType=off  TransfoNumber=1
  Trafo 70kV/20kV2 : spsThreePhaseTransformerTwoWindingsLib/Three-Phase Transformer (Two Windings)  Winding1Connection=Delta (D1)  Winding2Connection=Yg  CoreType=Three single-phase transformers  SetSaturation=off  Hysteresis=off  DataFile='hysteresis'  SetInitialFlux=off  Measurements=None  UNITS=pu  NominalPower=[ 250e6 , 50 ]  Winding1=[ 20e3 , 5e-3 , 0.1/(100*pi) ]  Winding2=[ 70e3 , 5e-3 , 0 ]  Rm=500  Lm=500  L0=0.5  Saturation=[ 0,0 ; 0.0024,1.2 ; 1.0,1.52 ]  InitialFluxes=[ 0.8 , -0.8 , 0.7 ]  BreakLoop=off  DiscreteSolver=Trapezoidal iterative  DataType=off  TransfoNumber=1
  Trafo 70kV/20kV3 : spsThreePhaseTransformerTwoWindingsLib/Three-Phase Transformer (Two Windings)  Winding1Connection=Delta (D1)  Winding2Connection=Yg  CoreType=Three single-phase transformers  SetSaturation=off  Hysteresis=off  DataFile='hysteresis'  SetInitialFlux=off  Measurements=None  UNITS=pu  NominalPower=[ 250e6 , 50 ]  Winding1=[ 20e3 , 5e-3 , 0.1/(100*pi) ]  Winding2=[ 70e3 , 5e-3 , 0 ]  Rm=500  Lm=500  L0=0.5  Saturation=[ 0,0 ; 0.0024,1.2 ; 1.0,1.52 ]  InitialFluxes=[ 0.8 , -0.8 , 0.7 ]  BreakLoop=off  DiscreteSolver=Trapezoidal iterative  DataType=off  TransfoNumber=1
  Trafo 70kV/230kV1 : spsThreePhaseTransformerTwoWindingsLib/Three-Phase Transformer (Two Windings)  Winding1Connection=Delta (D1)  Winding2Connection=Yg  CoreType=Three single-phase transformers  SetSaturation=off  Hysteresis=off  DataFile='hysteresis'  SetInitialFlux=off  Measurements=None  UNITS=pu  NominalPower=[ 250e6 , 50 ]  Winding1=[ 70e3 , 5e-3 , 0.1/(100*pi) ]  Winding2=[ 230e3 , 5e-3 , 0 ]  Rm=500  Lm=500  L0=0.5  Saturation=[ 0,0 ; 0.0024,1.2 ; 1.0,1.52 ]  InitialFluxes=[ 0.8 , -0.8 , 0.7 ]  BreakLoop=off  DiscreteSolver=Trapezoidal iterative  DataType=off  TransfoNumber=1
  Trafo 70kV/230kV2 : spsThreePhaseTransformerTwoWindingsLib/Three-Phase Transformer (Two Windings)  Winding1Connection=Delta (D1)  Winding2Connection=Yg  CoreType=Three single-phase transformers  SetSaturation=off  Hysteresis=off  DataFile='hysteresis'  SetInitialFlux=off  Measurements=None  UNITS=pu  NominalPower=[ 250e6 , 50 ]  Winding1=[ 70e3 , 5e-3 , 0.1/(100*pi) ]  Winding2=[ 230e3 , 5e-3 , 0 ]  Rm=500  Lm=500  L0=0.5  Saturation=[ 0,0 ; 0.0024,1.2 ; 1.0,1.52 ]  InitialFluxes=[ 0.8 , -0.8 , 0.7 ]  BreakLoop=off  DiscreteSolver=Trapezoidal iterative  DataType=off  TransfoNumber=1
  Trafo 70kV/230kV3 : spsThreePhaseTransformerTwoWindingsLib/Three-Phase Transformer (Two Windings)  Winding1Connection=Delta (D1)  Winding2Connection=Yg  CoreType=Three single-phase transformers  SetSaturation=off  Hysteresis=off  DataFile='hysteresis'  SetInitialFlux=off  Measurements=None  UNITS=pu  NominalPower=[ 250e6 , 50 ]  Winding1=[ 70e3 , 5e-3 , 0.1/(100*pi) ]  Winding2=[ 230e3 , 5e-3 , 0 ]  Rm=500  Lm=500  L0=0.5  Saturation=[ 0,0 ; 0.0024,1.2 ; 1.0,1.52 ]  InitialFluxes=[ 0.8 , -0.8 , 0.7 ]  BreakLoop=off  DiscreteSolver=Trapezoidal iterative  DataType=off  TransfoNumber=1
  UKM : spsThreePhaseParallelRLCLoadLib/Three-Phase Parallel RLC Load  LConnTagsString=A|B|C  Configuration=Y (grounded)  NominalVoltage=20e3  Vabc=[1e3 1e3 1e3]  Vabcp=[1e3 1e3 1e3]  NominalFrequency=50  UnbalancedPower=off  ActivePower=5.85e9  InductivePower=2.83e9  CapacitivePower=0  Pabc=[10e3 9e3 11e3]  QLabc=[100 90 110]  QCabc=[100 90 110]  Pabcp=[10e3 9e3 11e3]  QLabcp=[100 90 110]  QCabcp=[100 90 110]  Measurements=Branch voltages and currents  LoadType=constant Z
  Vref PLTA : Constant
  Vref PLTB : Constant
  Vref PLTP : Constant
  Vref PLTU : Constant
  powergui : spspowerguiLib/powergui  Priority=1  SimulationMode=Phasor  SampleTime=50e-6  frequency=50  Iterations=150  frequencyindice=50  Pbase=100e6  ErrMax=1e-4  UnitsV=kV  UnitsW=MW  buscounter=58  FunctionMessages=off  echomessages=off  EnableUseOfTLC=off  CurrentSourceSwitches=off  DisableSnubberDevices=off  DisableRonSwitches=off  DisableVfSwitches=off  DisplayEquations=off  AutomaticDiscreteSolvers=off  SolverType=Tustin/Backward Euler (TBE)  Interpol=off  ExternalGateDelay=off  methode=off  Ts=100  x0status=blocks  SPID=on  SwTol=0  HookPort=off  NonlinearTolerance=1e-4  nMaxIteration=100  ContinueOnMaxIteration=off  RestoreLinks=warning  ResistiveCurrentMeasurement=off  Frange=[0:2:500]  Ylog=off  Xlog=on  ShowGrid=off  save=off  variable=ZData  structure=0  ZoomFFT=off  StartTime=0.0  cycles=1  DisplayStyle=1  fundamental=60  FreqAxis=off  MaxFrequency=1000  frequencyindicesteady=1  RmsSteady=1  display=off
  wires:
  Pref PLTU/1 -> PLTU/1
  Excitation System PLTU/1 -> PLTU/2
  Vref PLTU/1 -> Excitation System PLTU/1
  PLTU/1 -> Bus Selector1/1
  Bus Selector1/2 -> Excitation System PLTU/2  "<Stator voltage  vd (pu)>"
  Bus Selector1/1 -> Excitation System PLTU/3  "<Stator voltage  vq (pu)>"
  PLTB/1 -> Bus Selector3/1
  Pref PLTB/1 -> PLTB/1
  Bus Selector3/1 -> Excitation System PLTB/3  "<Stator voltage  vq (pu)>"
  Excitation System PLTB/1 -> PLTB/2
  Bus Selector3/2 -> Excitation System PLTB/2  "<Stator voltage  vd (pu)>"
  Vref PLTB/1 -> Excitation System PLTB/1
  PLTA/1 -> Bus Selector2/1
  Pref PLTA/1 -> PLTA/1
  Bus Selector2/1 -> Excitation System PLTA/3  "<Stator voltage  vq (pu)>"
  Excitation System PLTA/1 -> PLTA/2
  Bus Selector2/2 -> Excitation System PLTA/2  "<Stator voltage  vd (pu)>"
  Vref PLTA/1 -> Excitation System PLTA/1
  "PLTP "/1 -> Bus Selector4/1
  Pref PLTP/1 -> "PLTP "/1
  Bus Selector4/1 -> Excitation System PLTP/3  "<Stator voltage  vq (pu)>"
  Excitation System PLTP/1 -> "PLTP "/2
  Bus Selector4/2 -> Excitation System PLTP/2  "<Stator voltage  vd (pu)>"
  Vref PLTP/1 -> Excitation System PLTP/1
  Multimeter/1 -> Scope/1
  connections:
  PLTU/RConn1 -- Three-Phase V-I Measurement1/LConn1
  PLTU/RConn2 -- Three-Phase V-I Measurement1/LConn2
  PLTU/RConn3 -- Three-Phase V-I Measurement1/LConn3
  PLTB/RConn3 -- Three-Phase V-I Measurement2/LConn3
  PLTB/RConn2 -- Three-Phase V-I Measurement2/LConn2
  PLTB/RConn1 -- Three-Phase V-I Measurement2/LConn1
  PLTA/RConn1 -- Pengukuran PLTA/LConn1
  PLTA/RConn2 -- Pengukuran PLTA/LConn2
  PLTA/RConn3 -- Pengukuran PLTA/LConn3
  "PLTP "/RConn1 -- Three-Phase V-I Measurement4/LConn1
  "PLTP "/RConn2 -- Three-Phase V-I Measurement4/LConn2
  "PLTP "/RConn3 -- Three-Phase V-I Measurement4/LConn3
  Three-Phase Breaker27/RConn1 -- 20kV/70kV/LConn1
  Three-Phase Breaker27/RConn2 -- 20kV/70kV/LConn2
  Three-Phase Breaker27/RConn3 -- 20kV/70kV/LConn3
  Three-Phase Breaker28/LConn1 -- 20kV/70kV/RConn1
  Three-Phase Breaker28/LConn2 -- 20kV/70kV/RConn2
  Three-Phase Breaker28/LConn3 -- 20kV/70kV/RConn3
  Three-Phase Breaker32/LConn1 -- 70kV/230kV/RConn1
  Three-Phase Breaker32/LConn2 -- 70kV/230kV/RConn2
  Three-Phase Breaker32/LConn3 -- 70kV/230kV/RConn3
  Three-Phase Breaker56/RConn1 -- 70kV/230kV/LConn1
  Three-Phase Breaker56/RConn2 -- 70kV/230kV/LConn2
  Three-Phase Breaker56/RConn3 -- 70kV/230kV/LConn3
  Three-Phase Breaker36/RConn1 -- "PLTP -- Gardu 1"/LConn1
  Three-Phase Breaker36/RConn2 -- "PLTP -- Gardu 1"/LConn2
  Three-Phase Breaker36/RConn3 -- "PLTP -- Gardu 1"/LConn3
  Three-Phase Breaker57/LConn1 -- "PLTP -- Gardu 1"/RConn1
  Three-Phase Breaker57/LConn2 -- "PLTP -- Gardu 1"/RConn2
  Three-Phase Breaker57/LConn3 -- "PLTP -- Gardu 1"/RConn3
  Three-Phase Breaker58/LConn3 -- "230kV/70kV "/RConn3
  Three-Phase Breaker59/RConn2 -- "230kV/70kV "/LConn2
  Three-Phase Breaker58/LConn1 -- "230kV/70kV "/RConn1
  Three-Phase Breaker59/RConn3 -- "230kV/70kV "/LConn3
  Three-Phase Breaker59/RConn1 -- "230kV/70kV "/LConn1
  Three-Phase Breaker58/LConn2 -- "230kV/70kV "/RConn2
  Trafo 230kV/70kV 1/RConn3 -- Three-Phase Breaker60/LConn3
  Trafo 20kV/70kV1/RConn1 -- Three-Phase Breaker29/LConn1
  Trafo 230kV/70kV 1/LConn3 -- Three-Phase Breaker61/RConn3
  Trafo 230kV/70kV 1/LConn2 -- Three-Phase Breaker61/RConn2
  Trafo 230kV/70kV 1/RConn2 -- Three-Phase Breaker60/LConn2
  Three-Phase Breaker37/RConn2 -- "Line PLTU -- Gardu 2"/LConn2
  Trafo 70kV/230kV1/RConn3 -- Three-Phase Breaker33/LConn3
  Trafo 20kV/70kV1/LConn3 -- Three-Phase Breaker26/RConn3
  Trafo 70kV/230kV1/LConn2 -- Three-Phase Breaker40/RConn2
  Trafo 20kV/70kV1/LConn2 -- Three-Phase Breaker26/RConn2
  Trafo 70kV/230kV1/LConn3 -- Three-Phase Breaker40/RConn3
  Trafo 70kV/230kV1/RConn1 -- Three-Phase Breaker33/LConn1
  Trafo 20kV/70kV1/LConn1 -- Three-Phase Breaker26/RConn1
  Trafo 70kV/230kV1/LConn1 -- Three-Phase Breaker40/RConn1
  Three-Phase Breaker41/LConn2 -- "Line PLTU -- Gardu 2"/RConn2
  Three-Phase Breaker37/RConn1 -- "Line PLTU -- Gardu 2"/LConn1
  Trafo 20kV/70kV1/RConn3 -- Three-Phase Breaker29/LConn3
  Trafo 20kV/70kV1/RConn2 -- Three-Phase Breaker29/LConn2
  Trafo 230kV/70kV 1/LConn1 -- Three-Phase Breaker61/RConn1
  Three-Phase Breaker41/LConn3 -- "Line PLTU -- Gardu 2"/RConn3
  Trafo 230kV/70kV 1/RConn1 -- Three-Phase Breaker60/LConn1
  Three-Phase Breaker41/LConn1 -- "Line PLTU -- Gardu 2"/RConn1
  Three-Phase Breaker37/RConn3 -- "Line PLTU -- Gardu 2"/LConn3
  Trafo 70kV/230kV1/RConn2 -- Three-Phase Breaker33/LConn2
  Trafo 230kV/70kV 2/RConn3 -- Three-Phase Breaker63/LConn3
  Trafo 20kV/70kV2/RConn1 -- Three-Phase Breaker30/LConn1
  Trafo 230kV/70kV 2/LConn3 -- Three-Phase Breaker64/RConn3
  Trafo 230kV/70kV 2/LConn2 -- Three-Phase Breaker64/RConn2
  Trafo 230kV/70kV 2/RConn2 -- Three-Phase Breaker63/LConn2
  Three-Phase Breaker38/RConn2 -- "Line PLTA -- Gardu 3"/LConn2
  Trafo 70kV/230kV2/RConn3 -- Three-Phase Breaker34/LConn3
  Trafo 20kV/70kV2/LConn3 -- Three-Phase Breaker24/RConn3
  Trafo 70kV/230kV2/LConn2 -- Three-Phase Breaker42/RConn2
  Trafo 20kV/70kV2/LConn2 -- Three-Phase Breaker24/RConn2
  Trafo 70kV/230kV2/LConn3 -- Three-Phase Breaker42/RConn3
  Trafo 70kV/230kV2/RConn1 -- Three-Phase Breaker34/LConn1
  Trafo 20kV/70kV2/LConn1 -- Three-Phase Breaker24/RConn1
  Trafo 70kV/230kV2/LConn1 -- Three-Phase Breaker42/RConn1
  Three-Phase Breaker62/LConn2 -- "Line PLTA -- Gardu 3"/RConn2
  Three-Phase Breaker38/RConn1 -- "Line PLTA -- Gardu 3"/LConn1
  Trafo 20kV/70kV2/RConn3 -- Three-Phase Breaker30/LConn3
  Trafo 20kV/70kV2/RConn2 -- Three-Phase Breaker30/LConn2
  Trafo 230kV/70kV 2/LConn1 -- Three-Phase Breaker64/RConn1
  Three-Phase Breaker62/LConn3 -- "Line PLTA -- Gardu 3"/RConn3
  Trafo 230kV/70kV 2/RConn1 -- Three-Phase Breaker63/LConn1
  Three-Phase Breaker62/LConn1 -- "Line PLTA -- Gardu 3"/RConn1
  Three-Phase Breaker38/RConn3 -- "Line PLTA -- Gardu 3"/LConn3
  Trafo 70kV/230kV2/RConn2 -- Three-Phase Breaker34/LConn2
  Trafo 230kV/70kV 3/RConn3 -- Three-Phase Breaker66/LConn3
  Trafo 20kV/70kV3/RConn1 -- Three-Phase Breaker31/LConn1
  Trafo 230kV/70kV 3/LConn3 -- Three-Phase Breaker67/RConn3
  Trafo 230kV/70kV 3/LConn2 -- Three-Phase Breaker67/RConn2
  Trafo 230kV/70kV 3/RConn2 -- Three-Phase Breaker66/LConn2
  Three-Phase Breaker39/RConn2 -- "Line PLTB -- Gardu 4"/LConn2
  Trafo 70kV/230kV3/RConn3 -- Three-Phase Breaker35/LConn3
  Trafo 20kV/70kV3/LConn3 -- Three-Phase Breaker25/RConn3
  Trafo 70kV/230kV3/LConn2 -- Three-Phase Breaker43/RConn2
  Trafo 20kV/70kV3/LConn2 -- Three-Phase Breaker25/RConn2
  Trafo 70kV/230kV3/LConn3 -- Three-Phase Breaker43/RConn3
  Trafo 70kV/230kV3/RConn1 -- Three-Phase Breaker35/LConn1
  Trafo 20kV/70kV3/LConn1 -- Three-Phase Breaker25/RConn1
  Trafo 70kV/230kV3/LConn1 -- Three-Phase Breaker43/RConn1
  Three-Phase Breaker65/LConn2 -- "Line PLTB -- Gardu 4"/RConn2
  Three-Phase Breaker39/RConn1 -- "Line PLTB -- Gardu 4"/LConn1
  Trafo 20kV/70kV3/RConn3 -- Three-Phase Breaker31/LConn3
  Trafo 20kV/70kV3/RConn2 -- Three-Phase Breaker31/LConn2
  Trafo 230kV/70kV 3/LConn1 -- Three-Phase Breaker67/RConn1
  Three-Phase Breaker65/LConn3 -- "Line PLTB -- Gardu 4"/RConn3
  Trafo 230kV/70kV 3/RConn1 -- Three-Phase Breaker66/LConn1
  Three-Phase Breaker65/LConn1 -- "Line PLTB -- Gardu 4"/RConn1
  Three-Phase Breaker39/RConn3 -- "Line PLTB -- Gardu 4"/LConn3
  Trafo 70kV/230kV3/RConn2 -- Three-Phase Breaker35/LConn2
  Three-Phase Breaker45/RConn3 -- "Gardu 1 -- Gardu 2"/LConn1
  Three-Phase Breaker45/RConn2 -- "Gardu 1 -- Gardu 2"/LConn2
  "Gardu 1 -- Gardu 2"/LConn3 -- Three-Phase Breaker45/RConn1
  "Gardu 1 -- Gardu 2"/RConn1 -- Three-Phase Breaker44/LConn3
  "Gardu 1 -- Gardu 2"/RConn2 -- Three-Phase Breaker44/LConn2
  "Gardu 1 -- Gardu 2"/RConn3 -- Three-Phase Breaker44/LConn1
  Three-Phase Breaker47/RConn3 -- "Gardu 1 -- Gardu 3"/LConn1
  "Gardu 1 -- Gardu 3"/RConn1 -- Three-Phase Breaker46/LConn3
  "Gardu 1 -- Gardu 3"/LConn3 -- Three-Phase Breaker47/RConn1
  "Gardu 1 -- Gardu 3"/RConn2 -- Three-Phase Breaker46/LConn2
  "Gardu 1 -- Gardu 3"/RConn3 -- Three-Phase Breaker46/LConn1
  Three-Phase Breaker47/RConn2 -- "Gardu 1 -- Gardu 3"/LConn2
  "Gardu 2 -- Gardu 3"/RConn1 -- Three-Phase Breaker50/LConn3
  "Gardu 2 -- Gardu 3"/LConn3 -- Three-Phase Breaker51/RConn1
  "Gardu 1 -- Gardu 4"/RConn2 -- Three-Phase Breaker48/LConn2
  Three-Phase Breaker49/RConn2 -- "Gardu 1 -- Gardu 4"/LConn2
  "Gardu 2 -- Gardu 3"/RConn2 -- Three-Phase Breaker50/LConn2
  "Gardu 2 -- Gardu 3"/RConn3 -- Three-Phase Breaker50/LConn1
  "Gardu 1 -- Gardu 4"/RConn1 -- Three-Phase Breaker48/LConn3
  "Gardu 1 -- Gardu 4"/RConn3 -- Three-Phase Breaker48/LConn1
  Three-Phase Breaker51/RConn2 -- "Gardu 2 -- Gardu 3"/LConn2
  "Gardu 1 -- Gardu 4"/LConn3 -- Three-Phase Breaker49/RConn1
  Three-Phase Breaker49/RConn3 -- "Gardu 1 -- Gardu 4"/LConn1
  Three-Phase Breaker51/RConn3 -- "Gardu 2 -- Gardu 3"/LConn1
  "Gardu 3 -- Gardu 4"/RConn1 -- Three-Phase Breaker54/LConn3
  "Gardu 3 -- Gardu 4"/LConn3 -- Three-Phase Breaker55/RConn1
  "Gardu 2 -- Gardu 4"/RConn2 -- Three-Phase Breaker52/LConn2
  Three-Phase Breaker53/RConn2 -- "Gardu 2 -- Gardu 4"/LConn2
  "Gardu 3 -- Gardu 4"/RConn2 -- Three-Phase Breaker54/LConn2
  "Gardu 3 -- Gardu 4"/RConn3 -- Three-Phase Breaker54/LConn1
  "Gardu 2 -- Gardu 4"/RConn1 -- Three-Phase Breaker52/LConn3
  "Gardu 2 -- Gardu 4"/RConn3 -- Three-Phase Breaker52/LConn1
  Three-Phase Breaker55/RConn2 -- "Gardu 3 -- Gardu 4"/LConn2
  "Gardu 2 -- Gardu 4"/LConn3 -- Three-Phase Breaker53/RConn1
  Three-Phase Breaker53/RConn3 -- "Gardu 2 -- Gardu 4"/LConn1
  Three-Phase Breaker55/RConn3 -- "Gardu 3 -- Gardu 4"/LConn1
  Trafo 70kV/20kV1/RConn3 -- Three-Phase Breaker70/LConn3
  Trafo 70kV/20kV1/RConn2 -- Three-Phase Breaker70/LConn2
  Trafo 70kV/20kV1/LConn3 -- Three-Phase Breaker71/RConn3
  Trafo 70kV/20kV1/RConn1 -- Three-Phase Breaker70/LConn1
  Trafo 70kV/20kV1/LConn1 -- Three-Phase Breaker71/RConn1
  Trafo 70kV/20kV1/LConn2 -- Three-Phase Breaker71/RConn2
  Trafo 70kV/20kV2/RConn3 -- Three-Phase Breaker72/LConn3
  Trafo 70kV/20kV2/RConn2 -- Three-Phase Breaker72/LConn2
  Trafo 70kV/20kV2/LConn3 -- Three-Phase Breaker73/RConn3
  Trafo 70kV/20kV2/RConn1 -- Three-Phase Breaker72/LConn1
  Trafo 70kV/20kV2/LConn1 -- Three-Phase Breaker73/RConn1
  Trafo 70kV/20kV2/LConn2 -- Three-Phase Breaker73/RConn2
  Three-Phase Breaker76/RConn1 -- 70kV/20kV/LConn1
  Three-Phase Breaker76/RConn3 -- 70kV/20kV/LConn3
  Three-Phase Breaker76/RConn2 -- 70kV/20kV/LConn2
  Three-Phase Breaker77/RConn1 -- "Gardu 1 -- RT"/LConn1
  Three-Phase Breaker77/RConn2 -- "Gardu 1 -- RT"/LConn2
  Three-Phase Breaker77/RConn3 -- "Gardu 1 -- RT"/LConn3
  Three-Phase Breaker78/LConn1 -- "Gardu 1 -- RT"/RConn1
  Three-Phase Breaker78/LConn2 -- "Gardu 1 -- RT"/RConn2
  Three-Phase Breaker78/LConn3 -- "Gardu 1 -- RT"/RConn3
  Three-Phase Breaker79/LConn2 -- 20kV/380V/RConn2
  Three-Phase Breaker79/LConn3 -- 20kV/380V/RConn3
  Three-Phase Breaker79/LConn1 -- 20kV/380V/RConn1
  Three-Phase Breaker103/LConn3 -- "Gardu 4 -- PubSos"/RConn3
  Three-Phase Breaker102/RConn2 -- "Gardu 4 -- PubSos"/LConn2
  Three-Phase Breaker103/LConn1 -- "Gardu 4 -- PubSos"/RConn1
  Three-Phase Breaker103/LConn2 -- "Gardu 4 -- PubSos"/RConn2
  Three-Phase Breaker102/RConn3 -- "Gardu 4 -- PubSos"/LConn3
  Trafo 20kV/380V1/RConn2 -- Three-Phase Breaker104/LConn2
  Trafo 70kV/20kV3/LConn2 -- Three-Phase Breaker101/RConn2
  Trafo 20kV/380V1/RConn3 -- Three-Phase Breaker104/LConn3
  Trafo 70kV/20kV3/LConn1 -- Three-Phase Breaker101/RConn1
  Trafo 70kV/20kV3/LConn3 -- Three-Phase Breaker101/RConn3
  Trafo 20kV/380V1/RConn1 -- Three-Phase Breaker104/LConn1
  Three-Phase Breaker102/RConn1 -- "Gardu 4 -- PubSos"/LConn1
  Three-Phase Breaker28/RConn1 -- Three-Phase Breaker56/LConn1
  Three-Phase Breaker28/RConn2 -- Three-Phase Breaker56/LConn2
  Three-Phase Breaker28/RConn3 -- Three-Phase Breaker56/LConn3
  Three-Phase Breaker58/RConn1 -- Three-Phase Breaker47/LConn1 -- Three-Phase Breaker76/LConn1 -- Three-Phase Breaker49/LConn1 -- Three-Phase Breaker45/LConn1
  Three-Phase Breaker58/RConn2 -- Three-Phase Breaker45/LConn2 -- Three-Phase Breaker47/LConn2 -- Three-Phase Breaker76/LConn2 -- Three-Phase Breaker49/LConn2
  Three-Phase Breaker58/RConn3 -- Three-Phase Breaker45/LConn3 -- Three-Phase Breaker47/LConn3 -- Three-Phase Breaker76/LConn3 -- Three-Phase Breaker49/LConn3
  Three-Phase Breaker29/RConn1 -- Three-Phase Breaker40/LConn1
  Three-Phase Breaker29/RConn2 -- Three-Phase Breaker40/LConn2
  Three-Phase Breaker29/RConn3 -- Three-Phase Breaker40/LConn3
  Three-Phase Breaker60/RConn1 -- Three-Phase Breaker44/RConn1 -- Three-Phase Breaker51/LConn1 -- Three-Phase Breaker53/LConn1 -- Three-Phase Breaker71/LConn1
  Three-Phase Breaker60/RConn2 -- Three-Phase Breaker44/RConn2 -- Three-Phase Breaker51/LConn2 -- Three-Phase Breaker53/LConn2 -- Three-Phase Breaker71/LConn2
  Three-Phase Breaker71/LConn3 -- Three-Phase Breaker53/LConn3 -- Three-Phase Breaker51/LConn3 -- Three-Phase Breaker44/RConn3 -- Three-Phase Breaker60/RConn3
  Three-Phase Breaker30/RConn1 -- Three-Phase Breaker42/LConn1
  Three-Phase Breaker30/RConn2 -- Three-Phase Breaker42/LConn2
  Three-Phase Breaker42/LConn3 -- Three-Phase Breaker30/RConn3
  Three-Phase Breaker63/RConn1 -- Three-Phase Breaker55/LConn1 -- Three-Phase Breaker73/LConn1 -- Three-Phase Breaker50/RConn1 -- Three-Phase Breaker46/RConn1
  Three-Phase Breaker63/RConn2 -- Three-Phase Breaker55/LConn2 -- Three-Phase Breaker73/LConn2 -- Three-Phase Breaker50/RConn2 -- Three-Phase Breaker46/RConn2
  Three-Phase Breaker63/RConn3 -- Three-Phase Breaker55/LConn3 -- Three-Phase Breaker73/LConn3 -- Three-Phase Breaker50/RConn3 -- Three-Phase Breaker46/RConn3
  Three-Phase Breaker31/RConn1 -- Three-Phase Breaker43/LConn1
  Three-Phase Breaker31/RConn2 -- Three-Phase Breaker43/LConn2
  Three-Phase Breaker31/RConn3 -- Three-Phase Breaker43/LConn3
  Three-Phase Breaker66/RConn1 -- Three-Phase Breaker101/LConn1 -- Three-Phase Breaker54/RConn1 -- Three-Phase Breaker52/RConn1 -- Three-Phase Breaker48/RConn1
  Three-Phase Breaker66/RConn2 -- Three-Phase Breaker101/LConn2 -- Three-Phase Breaker54/RConn2 -- Three-Phase Breaker52/RConn2 -- Three-Phase Breaker48/RConn2
  Three-Phase Breaker66/RConn3 -- Three-Phase Breaker101/LConn3 -- Three-Phase Breaker54/RConn3 -- Three-Phase Breaker52/RConn3 -- Three-Phase Breaker48/RConn3
  Three-Phase V-I Measurement4/RConn1 -- Three-Phase Breaker27/LConn1
  Three-Phase V-I Measurement4/RConn2 -- Three-Phase Breaker27/LConn2
  Three-Phase V-I Measurement4/RConn3 -- Three-Phase Breaker27/LConn3
  Three-Phase V-I Measurement1/RConn1 -- Three-Phase Breaker26/LConn1
  Three-Phase V-I Measurement1/RConn2 -- Three-Phase Breaker26/LConn2
  Three-Phase V-I Measurement1/RConn3 -- Three-Phase Breaker26/LConn3
  Pengukuran PLTA/RConn1 -- Three-Phase Breaker24/LConn1
  Pengukuran PLTA/RConn2 -- Three-Phase Breaker24/LConn2
  Pengukuran PLTA/RConn3 -- Three-Phase Breaker24/LConn3
  Three-Phase V-I Measurement2/RConn1 -- Three-Phase Breaker25/LConn1
  Three-Phase V-I Measurement2/RConn2 -- Three-Phase Breaker25/LConn2
  Three-Phase V-I Measurement2/RConn3 -- Three-Phase Breaker25/LConn3
  Three-Phase Breaker1/RConn3 -- "PLTP -- Gardu 1 (1)"/LConn3
  Three-Phase Breaker2/LConn3 -- "PLTP -- Gardu 1 (1)"/RConn3
  Three-Phase Breaker4/LConn3 -- "Line PLTU -- Gardu 1"/RConn3
  Three-Phase Breaker3/RConn3 -- "Line PLTU -- Gardu 1"/LConn3
  Three-Phase Breaker6/LConn3 -- "Line PLTA -- Gardu 1"/RConn3
  Three-Phase Breaker5/RConn3 -- "Line PLTA -- Gardu 1"/LConn3
  Three-Phase Breaker8/LConn3 -- "Line PLTB -- Gardu 1"/RConn3
  Three-Phase Breaker7/RConn3 -- "Line PLTB -- Gardu 1"/LConn3
  Three-Phase Breaker9/RConn2 -- "Gardu 1 -- RT1"/LConn2
  Three-Phase Breaker9/RConn3 -- "Gardu 1 -- RT1"/LConn3
  Three-Phase Breaker10/LConn2 -- "Gardu 1 -- RT1"/RConn2
  Three-Phase Breaker10/LConn3 -- "Gardu 1 -- RT1"/RConn3
  Three-Phase Breaker11/RConn3 -- "Gardu 4 -- PubSos1"/LConn3
  Three-Phase Breaker12/LConn3 -- "Gardu 4 -- PubSos1"/RConn3
  Three-Phase Breaker32/RConn1 -- Three-Phase Breaker36/LConn1 -- Three-Phase Breaker1/LConn1
  Three-Phase Breaker32/RConn2 -- Three-Phase Breaker36/LConn2 -- Three-Phase Breaker1/LConn2
  Three-Phase Breaker32/RConn3 -- Three-Phase Breaker1/LConn3 -- Three-Phase Breaker36/LConn3
  Three-Phase Breaker2/RConn1 -- Three-Phase Breaker57/RConn1 -- Three-Phase Breaker59/LConn1
  Three-Phase Breaker2/RConn2 -- Three-Phase Breaker57/RConn2 -- Three-Phase Breaker59/LConn2
  Three-Phase Breaker57/RConn3 -- Three-Phase Breaker2/RConn3 -- Three-Phase Breaker59/LConn3
  70kV/20kV/RConn1 -- Three-Phase Breaker77/LConn1
  Three-Phase Breaker77/LConn2 -- 70kV/20kV/RConn2
  Three-Phase Breaker77/LConn3 -- 70kV/20kV/RConn3
  20kV/380V/LConn1 -- Three-Phase Breaker78/RConn1
  20kV/380V/LConn2 -- Three-Phase Breaker78/RConn2
  20kV/380V/LConn3 -- Three-Phase Breaker78/RConn3
  Three-Phase Breaker37/LConn1 -- Three-Phase Breaker33/RConn1
  Three-Phase Breaker37/LConn2 -- Three-Phase Breaker33/RConn2
  Three-Phase Breaker37/LConn3 -- Three-Phase Breaker33/RConn3
  Three-Phase Breaker61/LConn1 -- Three-Phase Breaker41/RConn1
  Three-Phase Breaker61/LConn2 -- Three-Phase Breaker41/RConn2
  Three-Phase Breaker61/LConn3 -- Three-Phase Breaker41/RConn3
  Three-Phase Breaker102/LConn1 -- Trafo 70kV/20kV3/RConn1
  Three-Phase Breaker102/LConn2 -- Trafo 70kV/20kV3/RConn2
  Three-Phase Breaker102/LConn3 -- Trafo 70kV/20kV3/RConn3
  Trafo 20kV/380V1/LConn1 -- Three-Phase Breaker103/RConn1
  Trafo 20kV/380V1/LConn2 -- Three-Phase Breaker103/RConn2
  Trafo 20kV/380V1/LConn3 -- Three-Phase Breaker103/RConn3
  Three-Phase Breaker38/LConn1 -- Three-Phase Breaker34/RConn1
  Three-Phase Breaker38/LConn2 -- Three-Phase Breaker34/RConn2
  Three-Phase Breaker38/LConn3 -- Three-Phase Breaker34/RConn3
  Three-Phase Breaker64/LConn1 -- Three-Phase Breaker62/RConn1
  Three-Phase Breaker64/LConn2 -- Three-Phase Breaker62/RConn2
  Three-Phase Breaker64/LConn3 -- Three-Phase Breaker62/RConn3
  Three-Phase Breaker39/LConn1 -- Three-Phase Breaker35/RConn1
  Three-Phase Breaker39/LConn2 -- Three-Phase Breaker35/RConn2
  Three-Phase Breaker39/LConn3 -- Three-Phase Breaker35/RConn3
  Three-Phase Breaker67/LConn1 -- Three-Phase Breaker65/RConn1
  Three-Phase Breaker67/LConn2 -- Three-Phase Breaker65/RConn2
  Three-Phase Breaker67/LConn3 -- Three-Phase Breaker65/RConn3
  Three-Phase Breaker82/LConn1 -- Three-Phase Breaker79/RConn1 -- Three-Phase Breaker84/LConn1 -- Three-Phase Breaker83/LConn1 -- Three-Phase Breaker85/LConn1 -- Three-Phase Breaker86/LConn1
  Three-Phase Breaker82/LConn3 -- Three-Phase Breaker79/RConn3 -- Three-Phase Breaker84/LConn3 -- Three-Phase Breaker83/LConn3 -- Three-Phase Breaker85/LConn3 -- Three-Phase Breaker86/LConn3
  Three-Phase Breaker82/LConn2 -- Three-Phase Breaker79/RConn2 -- Three-Phase Breaker84/LConn2 -- Three-Phase Breaker83/LConn2 -- Three-Phase Breaker85/LConn2 -- Three-Phase Breaker86/LConn2
  Three-Phase Breaker84/RConn2 -- RT 3/LConn2
  Three-Phase Breaker82/RConn1 -- RT 1/LConn1
  Three-Phase Breaker82/RConn3 -- RT 1/LConn3
  Three-Phase Breaker85/RConn3 -- RT 4/LConn3
  Three-Phase Breaker85/RConn2 -- RT 4/LConn2
  Three-Phase Breaker85/RConn1 -- RT 4/LConn1
  Three-Phase Breaker84/RConn1 -- RT 3/LConn1
  Three-Phase Breaker82/RConn2 -- RT 1/LConn2
  Three-Phase Breaker84/RConn3 -- RT 3/LConn3
  Three-Phase Breaker86/RConn2 -- RT 5/LConn2
  Three-Phase Breaker86/RConn3 -- RT 5/LConn3
  Three-Phase Breaker86/RConn1 -- RT 5/LConn1
  Three-Phase Breaker89/LConn1 -- Three-Phase Breaker91/LConn1 -- Three-Phase Breaker70/RConn1 -- Three-Phase Breaker90/LConn1 -- Three-Phase Breaker87/LConn1 -- Three-Phase Breaker88/LConn1 -- Three-Phase Breaker92/LConn1
  Three-Phase Breaker90/LConn3 -- Three-Phase Breaker70/RConn3 -- Three-Phase Breaker88/LConn3 -- Three-Phase Breaker92/LConn3 -- Three-Phase Breaker89/LConn3 -- Three-Phase Breaker91/LConn3 -- Three-Phase Breaker87/LConn3
  Three-Phase Breaker91/LConn2 -- Three-Phase Breaker70/RConn2 -- Three-Phase Breaker87/LConn2 -- Three-Phase Breaker90/LConn2 -- Three-Phase Breaker92/LConn2 -- Three-Phase Breaker89/LConn2 -- Three-Phase Breaker88/LConn2
  Three-Phase Breaker92/RConn1 -- Mall & Hotel/LConn1
  Three-Phase Breaker88/RConn2 -- Industri Sedang/LConn2
  Three-Phase Breaker91/RConn1 -- Restoran & Toko/LConn1
  Three-Phase Breaker89/RConn2 -- Industri Besar/LConn2
  Three-Phase Breaker88/RConn1 -- Industri Sedang/LConn1
  Three-Phase Breaker90/RConn2 -- UKM/LConn2
  Three-Phase Breaker89/RConn1 -- Industri Besar/LConn1
  Three-Phase Breaker91/RConn2 -- Restoran & Toko/LConn2
  Three-Phase Breaker87/RConn1 -- Industri Kecil/LConn1
  Three-Phase Breaker90/RConn3 -- UKM/LConn3
  Three-Phase Breaker87/RConn3 -- Industri Kecil/LConn3
  Three-Phase Breaker87/RConn2 -- Industri Kecil/LConn2
  Three-Phase Breaker89/RConn3 -- Industri Besar/LConn3
  Three-Phase Breaker90/RConn1 -- UKM/LConn1
  Three-Phase Breaker92/RConn2 -- Mall & Hotel/LConn2
  Three-Phase Breaker88/RConn3 -- Industri Sedang/LConn3
  Three-Phase Breaker92/RConn3 -- Mall & Hotel/LConn3
  Three-Phase Breaker91/RConn3 -- Restoran & Toko/LConn3
  Three-Phase Breaker97/LConn3 -- Three-Phase Breaker94/LConn3 -- Three-Phase Breaker72/RConn3 -- Three-Phase Breaker95/LConn3 -- Three-Phase Breaker93/LConn3 -- Three-Phase Breaker96/LConn3
  Three-Phase Breaker97/LConn2 -- Three-Phase Breaker94/LConn2 -- Three-Phase Breaker72/RConn2 -- Three-Phase Breaker95/LConn2 -- Three-Phase Breaker93/LConn2 -- Three-Phase Breaker96/LConn2
  Three-Phase Breaker97/LConn1 -- Three-Phase Breaker94/LConn1 -- Three-Phase Breaker72/RConn1 -- Three-Phase Breaker95/LConn1 -- Three-Phase Breaker93/LConn1 -- Three-Phase Breaker96/LConn1
  Three-Phase Breaker94/RConn1 -- Pusat Server Data/LConn1
  Three-Phase Breaker93/RConn1 -- Rumah Sakit/LConn1
  Three-Phase Breaker94/RConn3 -- Pusat Server Data/LConn3
  Three-Phase Breaker95/RConn2 -- Kantor Lembaga Negara/LConn2
  Three-Phase Breaker95/RConn3 -- Kantor Lembaga Negara/LConn3
  Three-Phase Breaker95/RConn1 -- Kantor Lembaga Negara/LConn1
  Three-Phase Breaker96/RConn2 -- Istana Negara/LConn2
  Three-Phase Breaker96/RConn1 -- Istana Negara/LConn1
  Three-Phase Breaker93/RConn2 -- Rumah Sakit/LConn2
  Three-Phase Breaker97/RConn1 -- Pangkalan Militer/LConn1
  Three-Phase Breaker97/RConn2 -- Pangkalan Militer/LConn2
  Three-Phase Breaker93/RConn3 -- Rumah Sakit/LConn3
  Three-Phase Breaker96/RConn3 -- Istana Negara/LConn3
  Three-Phase Breaker94/RConn2 -- Pusat Server Data/LConn2
  Three-Phase Breaker97/RConn3 -- Pangkalan Militer/LConn3
  Three-Phase Breaker99/LConn1 -- Three-Phase Breaker104/RConn1 -- Three-Phase Breaker98/LConn1 -- Three-Phase Breaker100/LConn1
  Three-Phase Breaker99/LConn2 -- Three-Phase Breaker104/RConn2 -- Three-Phase Breaker98/LConn2 -- Three-Phase Breaker100/LConn2
  Three-Phase Breaker100/LConn3 -- Three-Phase Breaker99/LConn3 -- Three-Phase Breaker104/RConn3 -- Three-Phase Breaker98/LConn3
  Three-Phase Breaker98/RConn2 -- Rumah Ibadah/LConn2
  Three-Phase Breaker99/RConn3 -- Sekolah & Universitas/LConn3
  Penerangan Jalan Umum/LConn1 -- Three-Phase Breaker100/RConn1
  Penerangan Jalan Umum/LConn3 -- Three-Phase Breaker100/RConn3
  Three-Phase Breaker98/RConn1 -- Rumah Ibadah/LConn1
  Three-Phase Breaker99/RConn1 -- Sekolah & Universitas/LConn1
  Three-Phase Breaker98/RConn3 -- Rumah Ibadah/LConn3
  Three-Phase Breaker99/RConn2 -- Sekolah & Universitas/LConn2
  Penerangan Jalan Umum/LConn2 -- Three-Phase Breaker100/RConn2
